simulink model "scale_model_model_control"  (R2024b)
settings: Solver=VariableStepAuto  StartTime=0.0  StopTime=100  MaxStep=0.02  RelTol=1e-3
values from neighbouring files (symbols this model uses):
  A_adrcl = [zeros(N, 1)  eye(N, N) ... (first row only)    [init_scale_blade_suspended_control.m]
  A_ESO_d = [1-l1_ESO_d, delta_t-l1_ESO_d*delta_t, 1/2 * delta_t^2 - 1/2 * l1_ESO_d*delta_t^2 ... (first row only)    [init_scale_blade_suspended_control.m]
  A_MESO_d = A_o_d - l_MESO_d*C_o_d*A_o_d    [init_scale_blade_suspended_control.m]
  b0 = 1.025    [init_scale_blade_suspended_control.m]
  b_adrcl = [zeros(N-1, 1) ... (first row only)    [init_scale_blade_suspended_control.m]
  b_ESO_d = [1/2*b0*delta_t^2 - l1_ESO_d*b0*delta_t^2 ... (first row only)    [init_scale_blade_suspended_control.m]
  B_MESO_d = B_o_d - l_MESO_d*C_o_d*B_o_d    [init_scale_blade_suspended_control.m]
  c_t = [1, zeros(1, N)]    [init_scale_blade_suspended_control.m]
  delta_t = 0.01    [init_scale_blade_suspended_control.m]
  DLADRC_max_effort = 30    [init_scale_blade_suspended_control.m]
  DLQRMADRC_max_effort = 30    [init_scale_blade_suspended_control.m]
  eta_s_init_n = [p_s_init_n;Theta_s_init_n]    [init_scale_blade_suspended_control.m]
  g = 9.81    [init_scale_blade_suspended_control.m]
  inv_M_s = inv(M_s)    [init_scale_blade_suspended_control.m]
  k = ones(N,1)    [init_scale_blade_suspended_control.m]
  k1_c_d = (1 - z_cl)^2/delta_t^2    [init_scale_blade_suspended_control.m]
  k_c_T_dlqr = dlqr(A_m_dlqr,b_m_dlqr,Q,R)    [init_scale_blade_suspended_control.m]
  k_d_T_lqr = (e_m*c_T_d_m_lqr) \ b_m_lqr    [init_scale_blade_suspended_control.m]
  k_s_lqr = -inv(c_T_m_lqr*inv(A_m_lqr-b_m_lqr*k_c_T_lqr)*b_m_lqr)    [init_scale_blade_suspended_control.m]
  k_T_d = [k1_c_d, k2_c_d]    [init_scale_blade_suspended_control.m]
  k_w1_s = gamma * EA/lw1_s_init    (= 19634.9540849)    [init_scale_blade_suspended_control.m]
  k_w2_s = k_w1_s    (= 19634.9540849)    [init_scale_blade_suspended_control.m]
  L = 0.8    [init_scale_blade_suspended_control.m]
  l = ones(N+1, 1)    [init_scale_blade_suspended_control.m]
  l_ESO_d = [l1_ESO_d, l2_ESO_d, l3_ESO_d]'    [init_scale_blade_suspended_control.m]
  l_MESO_d = acker(A_o_d',C_o_d',[z_MESO,z_MESO,z_MESO])'    [init_scale_blade_suspended_control.m]
  lw1_s_init = tot_liftWire-0.14    (= 0.56)    [init_scale_blade_suspended_control.m]
  lw2_s = norm(p_h_s_init- posSling_s_n(:,1))-elong_lw2_s    [init_scale_blade_suspended_control.m]
  m_h_s = 0.01    [init_scale_blade_suspended_control.m]
  meanWSP = 1    [init_scale_blade_suspended_control.m]
  N = 2    [init_scale_blade_suspended_control.m]
  nu_s_init_b = zeros(6,1)    [init_scale_blade_suspended_control.m]
  p_h_dot_s_init = [0;0;0]    [init_scale_blade_suspended_control.m]
  p_h_s_init = posCraneTip_s + [0;0;lw1_s_init + elong_mainlw_s]    [init_scale_blade_suspended_control.m]
  posCOG_s = [0;0;0]    [init_scale_blade_suspended_control.m]
  posCraneTip_s = [0;0;-1.2]    [init_scale_blade_suspended_control.m]
  posSling_s_b = [posCOG_s + [slings_p1_new(1); -0.05; slings_p1_new(2)],                posCOG_s + [slings_p1_new(1); 0.05; slings_p1_new(2)],               posCOG_s + [slings_p2_new(1); -0.05; slings_p2_new(2)],               posCOG_s + [slings_p2_new(1); 0.05; slings_p2_new(2)]]    [init_scale_blade_suspended_control.m]
  posThruster_s_b = [posCOG_s + [0.03; 0.21; -0.05],                posCOG_s + [0.03; -0.21; -0.05],               posCOG_s + [0; 0.1825; -0.05],               posCOG_s + [0; -0.1825; -0.05]]    [init_scale_blade_suspended_control.m]
  totalMass_s = 0.391    [init_scale_blade_suspended_control.m]
  W = 0.05    [init_scale_blade_suspended_control.m]
undefined symbols (not defined in the file or in its folder): A_o_dlqr, b_o_dlqr, c_o_T_dlqr, k_o_lqr, linsys_v2, sigbuilder_block
libraries: MarIn_blade x104, simulink_extras x28, slpidlib x5, simulink x4
(part 3 of 3)

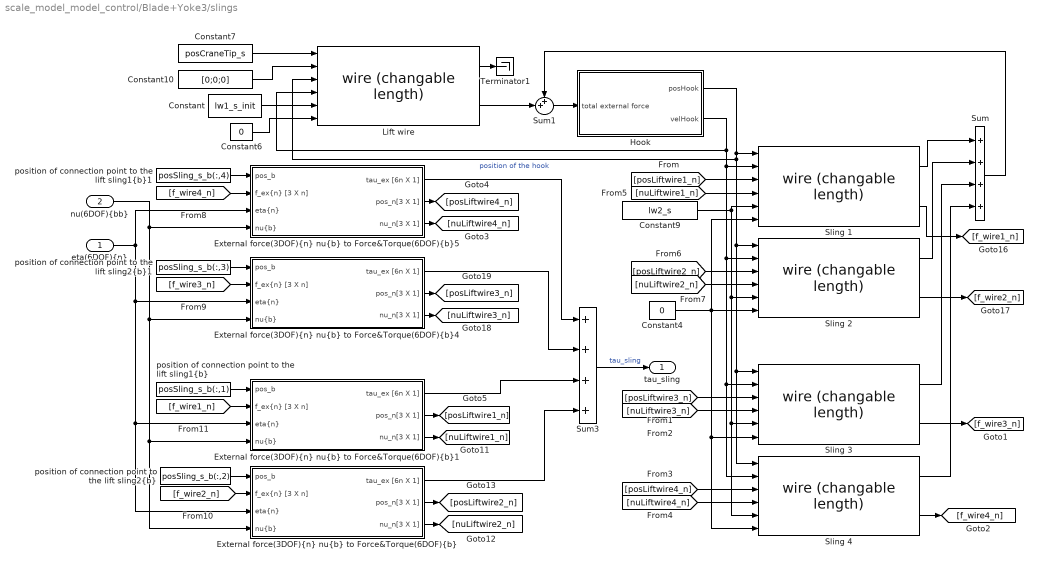
== system scale_model_model_control/Blade+Yoke3/slings ==
  "eta(6DOF){n}" : Inport
  "nu(6DOF){bb}" : Inport  Port=2
  Constant : Constant  Value=lw1_s_init
  Constant10 : Constant  Value=[0;0;0]
  Constant4 : Constant  Value=0
  Constant6 : Constant  Value=0
  Constant7 : Constant  Value=posCraneTip_s
  Constant9 : Constant  Value=lw2_s
  "External force(3DOF){n} nu{b} to Force&Torque(6DOF){b}" : Subsystem  AncestorBlock=MarIn_blade/Basic functions/External force(3DOF){n} nu{b} to Force&Torque(6DOF){b}  mask(External force(3DOF){n} nu{b} to Force&Torque(6DOF){b}){}
      mask help:
      | Translate position and velocity in {b} to {n}.
      |
      |
      | Author: Zhengru Ren
      | Date: April 22, 2017
  "External force(3DOF){n} nu{b} to Force&Torque(6DOF){b}1" : Subsystem  AncestorBlock=MarIn_blade/Basic functions/External force(3DOF){n} nu{b} to Force&Torque(6DOF){b}  mask(External force(3DOF){n} nu{b} to Force&Torque(6DOF){b}){}
      mask help:
      | Translate position and velocity in {b} to {n}.
      |
      |
      | Author: Zhengru Ren
      | Date: April 22, 2017
  "External force(3DOF){n} nu{b} to Force&Torque(6DOF){b}4" : Subsystem  AncestorBlock=MarIn_blade/Basic functions/External force(3DOF){n} nu{b} to Force&Torque(6DOF){b}  mask(External force(3DOF){n} nu{b} to Force&Torque(6DOF){b}){}
      mask help:
      | Translate position and velocity in {b} to {n}.
      |
      |
      | Author: Zhengru Ren
      | Date: April 22, 2017
  "External force(3DOF){n} nu{b} to Force&Torque(6DOF){b}5" : Subsystem  AncestorBlock=MarIn_blade/Basic functions/External force(3DOF){n} nu{b} to Force&Torque(6DOF){b}  mask(External force(3DOF){n} nu{b} to Force&Torque(6DOF){b}){}
      mask help:
      | Translate position and velocity in {b} to {n}.
      |
      |
      | Author: Zhengru Ren
      | Date: April 22, 2017
  Hook : Subsystem  AncestorBlock=|  mask(Hook){m_h=m_h_s, p_h_init=p_h_s_init, p_h_dot_init=p_h_dot_s_init}
      | MarIn_blade/Lifting equipments
      | (winch, wire, hook)/Hook
      mask prompts: m_h "Hook mass (m_h) [kg]"; p_h_init "Initial position of the hook"; p_h_dot_init "Initial velocity of the hook"
      mask help:
      | Used to simulate a hook.
      |
      | Author: Zhengru Ren
      | Date: May 20, 2016
      mask init:
      | invM_h = diag([1/m_h,1/m_h,1/m_h]);
  Lift wire : MarIn_blade/Lifting equipments (winch, wire, hook)/wire (changable length)  k=k_w1_s  c=d_w1_s
      settings: SourceProductName=MarIn (Blade)
  Sling {1..4} (4 alike) : MarIn_blade/Lifting equipments (winch, wire, hook)/wire (changable length)  k=k_w2_s  c=d_w2_s
      settings: SourceProductName=MarIn (Blade)
  Sum : Sum  Inputs=++++
  Sum1 : Sum  Inputs=++|
  Sum3 : Sum  Inputs=4
  Terminator1 : Terminator
  "position of connection point to the lift sling1{b}" : Constant  Value=posSling_s_b(:,1)
  "position of connection point to the lift sling1{b}1" : Constant  Value=posSling_s_b(:,4)
  "position of connection point to the lift sling2{b}" : Constant  Value=posSling_s_b(:,2)
  "position of connection point to the lift sling2{b}1" : Constant  Value=posSling_s_b(:,3)
  tau_sling : Outport
  wires:
  "nu(6DOF){bb}"/1 -> "External force(3DOF){n} nu{b} to Force&Torque(6DOF){b}"/4("nu{b}"), "External force(3DOF){n} nu{b} to Force&Torque(6DOF){b}1"/4("nu{b}"), "External force(3DOF){n} nu{b} to Force&Torque(6DOF){b}4"/4("nu{b}"), "External force(3DOF){n} nu{b} to Force&Torque(6DOF){b}5"/4("nu{b}")
  "position of connection point to the lift sling1{b}1"/1 -> "External force(3DOF){n} nu{b} to Force&Torque(6DOF){b}5"/1(pos_b)
  "External force(3DOF){n} nu{b} to Force&Torque(6DOF){b}"/1(tau_ex [6n X 1]) -> Sum3/4
  "eta(6DOF){n}"/1 -> "External force(3DOF){n} nu{b} to Force&Torque(6DOF){b}5"/3("eta{n}"), "External force(3DOF){n} nu{b} to Force&Torque(6DOF){b}"/3("eta{n}"), "External force(3DOF){n} nu{b} to Force&Torque(6DOF){b}1"/3("eta{n}"), "External force(3DOF){n} nu{b} to Force&Torque(6DOF){b}4"/3("eta{n}")
  "External force(3DOF){n} nu{b} to Force&Torque(6DOF){b}5"/1(tau_ex [6n X 1]) -> Sum3/1
  "position of connection point to the lift sling2{b}"/1 -> "External force(3DOF){n} nu{b} to Force&Torque(6DOF){b}"/1(pos_b)
  Sum3/1 -> tau_sling/1  "tau_sling"
  "External force(3DOF){n} nu{b} to Force&Torque(6DOF){b}4"/1(tau_ex [6n X 1]) -> Sum3/2
  [f_wire4_n] -> "External force(3DOF){n} nu{b} to Force&Torque(6DOF){b}5"/2("f_ex{n} [3 X n]")
  [f_wire3_n] -> "External force(3DOF){n} nu{b} to Force&Torque(6DOF){b}4"/2("f_ex{n} [3 X n]")
  "position of connection point to the lift sling2{b}1"/1 -> "External force(3DOF){n} nu{b} to Force&Torque(6DOF){b}4"/1(pos_b)
  "External force(3DOF){n} nu{b} to Force&Torque(6DOF){b}1"/3(nu_n[3 X 1]) -> [nuLiftwire1_n]
  "External force(3DOF){n} nu{b} to Force&Torque(6DOF){b}4"/2(pos_n[3 X 1]) -> [posLiftwire3_n]
  "position of connection point to the lift sling1{b}"/1 -> "External force(3DOF){n} nu{b} to Force&Torque(6DOF){b}1"/1(pos_b)
  "External force(3DOF){n} nu{b} to Force&Torque(6DOF){b}4"/3(nu_n[3 X 1]) -> [nuLiftwire3_n]
  [f_wire2_n] -> "External force(3DOF){n} nu{b} to Force&Torque(6DOF){b}"/2("f_ex{n} [3 X n]")
  "External force(3DOF){n} nu{b} to Force&Torque(6DOF){b}"/3(nu_n[3 X 1]) -> [nuLiftwire2_n]
  "External force(3DOF){n} nu{b} to Force&Torque(6DOF){b}"/2(pos_n[3 X 1]) -> [posLiftwire2_n]
  "External force(3DOF){n} nu{b} to Force&Torque(6DOF){b}1"/1(tau_ex [6n X 1]) -> Sum3/3
  "External force(3DOF){n} nu{b} to Force&Torque(6DOF){b}1"/2(pos_n[3 X 1]) -> [posLiftwire1_n]
  [f_wire1_n] -> "External force(3DOF){n} nu{b} to Force&Torque(6DOF){b}1"/2("f_ex{n} [3 X n]")
  Sling 4/2 -> [f_wire4_n]
  Sling 3/2 -> [f_wire3_n]
  Sling 4/1 -> Sum/4
  Sling 3/1 -> Sum/3
  [posLiftwire3_n] -> Sling 3/3
  [nuLiftwire3_n] -> Sling 3/4
  Hook/2(velHook) -> Sling 3/2, Sling 4/2, Sling 2/2, Sling 1/2, Lift wire/4
  Constant/1 -> Lift wire/5
  [posLiftwire1_n] -> Sling 1/3
  Sling 1/2 -> [f_wire1_n]
  [nuLiftwire1_n] -> Sling 1/4
  Sling 2/1 -> Sum/2
  Sling 2/2 -> [f_wire2_n]
  [posLiftwire2_n] -> Sling 2/3
  [nuLiftwire2_n] -> Sling 2/4
  Constant9/1 -> Sling 1/5, Sling 2/5, Sling 3/5, Sling 4/5
  Constant7/1 -> Lift wire/1
  Constant10/1 -> Lift wire/2
  Sum/1 -> Sum1/1
  Lift wire/2 -> Sum1/2
  Lift wire/1 -> Terminator1/1
  Sum1/1 -> Hook/1(total external force)
  Hook/1(posHook) -> Sling 3/1, Sling 4/1, Sling 2/1, Lift wire/3, Sling 1/1  "position of the hook"
  Constant4/1 -> Sling 2/6, Sling 1/6, Sling 3/6, Sling 4/6
  Constant6/1 -> Lift wire/6
  Sling 1/1 -> Sum/1
  [nuLiftwire4_n] -> Sling 4/4
  [posLiftwire4_n] -> Sling 4/3
  "External force(3DOF){n} nu{b} to Force&Torque(6DOF){b}5"/3(nu_n[3 X 1]) -> [nuLiftwire4_n]
  "External force(3DOF){n} nu{b} to Force&Torque(6DOF){b}5"/2(pos_n[3 X 1]) -> [posLiftwire4_n]

== system scale_model_model_control/Blade+Yoke3/thrusters ==
  "F_thrusters {b}" : Inport
  Demux : Demux
  Force(3DOF){b}2Force&Torque(6DOF){b}{,1..3} (4 alike) : MarIn_blade/Basic functions/Force(3DOF){b}2Force&Torque(6DOF){b}  posCOG_bb=posCOG_s
      settings: SourceProductName=MarIn (Blade)
  Sum3 : Sum  Inputs=4
  "position of connection point to thruster1{b}" : Constant  Value=posThruster_s_b(:,1)
  "position of connection point to thruster2{b}" : Constant  Value=posThruster_s_b(:,2)
  "position of connection point to thruster3{b}" : Constant  Value=posThruster_s_b(:,3)
  "position of connection point to thruster4{b}" : Constant  Value=posThruster_s_b(:,4)
  tau_thrusters : Outport
  wires:
  "position of connection point to thruster1{b}"/1 -> "Force(3DOF){b}2Force&Torque(6DOF){b}1"/1
  "position of connection point to thruster3{b}"/1 -> "Force(3DOF){b}2Force&Torque(6DOF){b}2"/1
  Sum3/1 -> tau_thrusters/1  "tau_thrusters"
  "position of connection point to thruster2{b}"/1 -> "Force(3DOF){b}2Force&Torque(6DOF){b}"/1
  "Force(3DOF){b}2Force&Torque(6DOF){b}"/1 -> Sum3/4
  "position of connection point to thruster4{b}"/1 -> "Force(3DOF){b}2Force&Torque(6DOF){b}3"/1
  "Force(3DOF){b}2Force&Torque(6DOF){b}3"/1 -> Sum3/1
  "Force(3DOF){b}2Force&Torque(6DOF){b}2"/1 -> Sum3/2
  "Force(3DOF){b}2Force&Torque(6DOF){b}1"/1 -> Sum3/3
  "F_thrusters {b}"/1 -> Demux/1
  Demux/4 -> "Force(3DOF){b}2Force&Torque(6DOF){b}3"/2
  Demux/3 -> "Force(3DOF){b}2Force&Torque(6DOF){b}2"/2
  Demux/1 -> "Force(3DOF){b}2Force&Torque(6DOF){b}1"/2
  Demux/2 -> "Force(3DOF){b}2Force&Torque(6DOF){b}"/2

== system scale_model_model_control/Blade+Yoke/slings/External force(3DOF){n} nu{b} to Force&Torque(6DOF){b} ==
  pos_b : Inport
  "f_ex{n} [3 X n]" : Inport  Port=2
  "eta{n}" : Inport  Port=3
  "nu{b}" : Inport  Port=4
  "Force(3DOF){b}2Force&Torque(6DOF){b}" : MarIn_blade/Basic functions/Force(3DOF){b}2Force&Torque(6DOF){b}  posCOG_bb=posCOG_s
      settings: SourceProductName=MarIn (Blade)
  "Translate velocity&force {n}2{b}" : MarIn_blade/Basic functions/Translate velocity&force {n}2{b}
      settings: SourceProductName=MarIn (Blade)
  "pos{b} nu{b} to pos{n}" : MarIn_blade/Basic functions/pos{b} nu{b} to pos{n}  posCOG_bb=posCOG_s
      settings: SourceProductName=MarIn (Blade)
  tau_ex [6n X 1] : Outport
  pos_n[3 X 1] : Outport  Port=2
  nu_n[3 X 1] : Outport  Port=3
  wires:
  "eta{n}"/1 -> "Translate velocity&force {n}2{b}"/1, "pos{b} nu{b} to pos{n}"/2
  "f_ex{n} [3 X n]"/1 -> "Translate velocity&force {n}2{b}"/2
  "Force(3DOF){b}2Force&Torque(6DOF){b}"/1 -> tau_ex [6n X 1]/1
  "Translate velocity&force {n}2{b}"/1 -> "Force(3DOF){b}2Force&Torque(6DOF){b}"/2  "External force{bb}"
  pos_b/1 -> "Force(3DOF){b}2Force&Torque(6DOF){b}"/1, "pos{b} nu{b} to pos{n}"/1
  "pos{b} nu{b} to pos{n}"/1 -> pos_n[3 X 1]/1
  "nu{b}"/1 -> "pos{b} nu{b} to pos{n}"/3
  "pos{b} nu{b} to pos{n}"/2 -> nu_n[3 X 1]/1

== system scale_model_model_control/Blade+Yoke/slings/External force(3DOF){n} nu{b} to Force&Torque(6DOF){b}1 ==
  pos_b : Inport
  "f_ex{n} [3 X n]" : Inport  Port=2
  "eta{n}" : Inport  Port=3
  "nu{b}" : Inport  Port=4
  "Force(3DOF){b}2Force&Torque(6DOF){b}" : MarIn_blade/Basic functions/Force(3DOF){b}2Force&Torque(6DOF){b}  posCOG_bb=posCOG_s
      settings: SourceProductName=MarIn (Blade)
  "Translate velocity&force {n}2{b}" : MarIn_blade/Basic functions/Translate velocity&force {n}2{b}
      settings: SourceProductName=MarIn (Blade)
  "pos{b} nu{b} to pos{n}" : MarIn_blade/Basic functions/pos{b} nu{b} to pos{n}  posCOG_bb=posCOG_s
      settings: SourceProductName=MarIn (Blade)
  tau_ex [6n X 1] : Outport
  pos_n[3 X 1] : Outport  Port=2
  nu_n[3 X 1] : Outport  Port=3
  wires:
  "eta{n}"/1 -> "Translate velocity&force {n}2{b}"/1, "pos{b} nu{b} to pos{n}"/2
  "f_ex{n} [3 X n]"/1 -> "Translate velocity&force {n}2{b}"/2
  "Force(3DOF){b}2Force&Torque(6DOF){b}"/1 -> tau_ex [6n X 1]/1
  "Translate velocity&force {n}2{b}"/1 -> "Force(3DOF){b}2Force&Torque(6DOF){b}"/2  "External force{bb}"
  pos_b/1 -> "Force(3DOF){b}2Force&Torque(6DOF){b}"/1, "pos{b} nu{b} to pos{n}"/1
  "pos{b} nu{b} to pos{n}"/1 -> pos_n[3 X 1]/1
  "nu{b}"/1 -> "pos{b} nu{b} to pos{n}"/3
  "pos{b} nu{b} to pos{n}"/2 -> nu_n[3 X 1]/1

== system scale_model_model_control/Blade+Yoke/slings/External force(3DOF){n} nu{b} to Force&Torque(6DOF){b}4 ==
  pos_b : Inport
  "f_ex{n} [3 X n]" : Inport  Port=2
  "eta{n}" : Inport  Port=3
  "nu{b}" : Inport  Port=4
  "Force(3DOF){b}2Force&Torque(6DOF){b}" : MarIn_blade/Basic functions/Force(3DOF){b}2Force&Torque(6DOF){b}  posCOG_bb=posCOG_s
      settings: SourceProductName=MarIn (Blade)
  "Translate velocity&force {n}2{b}" : MarIn_blade/Basic functions/Translate velocity&force {n}2{b}
      settings: SourceProductName=MarIn (Blade)
  "pos{b} nu{b} to pos{n}" : MarIn_blade/Basic functions/pos{b} nu{b} to pos{n}  posCOG_bb=posCOG_s
      settings: SourceProductName=MarIn (Blade)
  tau_ex [6n X 1] : Outport
  pos_n[3 X 1] : Outport  Port=2
  nu_n[3 X 1] : Outport  Port=3
  wires:
  "eta{n}"/1 -> "Translate velocity&force {n}2{b}"/1, "pos{b} nu{b} to pos{n}"/2
  "f_ex{n} [3 X n]"/1 -> "Translate velocity&force {n}2{b}"/2
  "Force(3DOF){b}2Force&Torque(6DOF){b}"/1 -> tau_ex [6n X 1]/1
  "Translate velocity&force {n}2{b}"/1 -> "Force(3DOF){b}2Force&Torque(6DOF){b}"/2  "External force{bb}"
  pos_b/1 -> "Force(3DOF){b}2Force&Torque(6DOF){b}"/1, "pos{b} nu{b} to pos{n}"/1
  "pos{b} nu{b} to pos{n}"/1 -> pos_n[3 X 1]/1
  "nu{b}"/1 -> "pos{b} nu{b} to pos{n}"/3
  "pos{b} nu{b} to pos{n}"/2 -> nu_n[3 X 1]/1

== system scale_model_model_control/Blade+Yoke/slings/External force(3DOF){n} nu{b} to Force&Torque(6DOF){b}5 ==
  pos_b : Inport
  "f_ex{n} [3 X n]" : Inport  Port=2
  "eta{n}" : Inport  Port=3
  "nu{b}" : Inport  Port=4
  "Force(3DOF){b}2Force&Torque(6DOF){b}" : MarIn_blade/Basic functions/Force(3DOF){b}2Force&Torque(6DOF){b}  posCOG_bb=posCOG_s
      settings: SourceProductName=MarIn (Blade)
  "Translate velocity&force {n}2{b}" : MarIn_blade/Basic functions/Translate velocity&force {n}2{b}
      settings: SourceProductName=MarIn (Blade)
  "pos{b} nu{b} to pos{n}" : MarIn_blade/Basic functions/pos{b} nu{b} to pos{n}  posCOG_bb=posCOG_s
      settings: SourceProductName=MarIn (Blade)
  tau_ex [6n X 1] : Outport
  pos_n[3 X 1] : Outport  Port=2
  nu_n[3 X 1] : Outport  Port=3
  wires:
  "eta{n}"/1 -> "Translate velocity&force {n}2{b}"/1, "pos{b} nu{b} to pos{n}"/2
  "f_ex{n} [3 X n]"/1 -> "Translate velocity&force {n}2{b}"/2
  "Force(3DOF){b}2Force&Torque(6DOF){b}"/1 -> tau_ex [6n X 1]/1
  "Translate velocity&force {n}2{b}"/1 -> "Force(3DOF){b}2Force&Torque(6DOF){b}"/2  "External force{bb}"
  pos_b/1 -> "Force(3DOF){b}2Force&Torque(6DOF){b}"/1, "pos{b} nu{b} to pos{n}"/1
  "pos{b} nu{b} to pos{n}"/1 -> pos_n[3 X 1]/1
  "nu{b}"/1 -> "pos{b} nu{b} to pos{n}"/3
  "pos{b} nu{b} to pos{n}"/2 -> nu_n[3 X 1]/1

== system scale_model_model_control/Blade+Yoke/slings/Hook ==
  total external force : Inport
  Integrator2 : Integrator  InitialCondition=p_h_dot_init  ContinuousStateAttributes='nu_hook'
  Integrator3 : Integrator  InitialCondition=p_h_init  ContinuousStateAttributes='pos_hook'
  Sum6 : Sum
  hook gravity : Constant  Value=[0;0;m_h*g]
  invM_h : Gain  Gain=invM_h  Multiplication=Matrix(K*u)
  posHook : Outport
  velHook : Outport  Port=2
  wires:
  Integrator2/1 -> velHook/1, Integrator3/1  "p_h_dot"
  total external force/1 -> Sum6/1
  hook gravity/1 -> Sum6/2
  invM_h/1 -> Integrator2/1  "p_h_ddot"
  Sum6/1 -> invM_h/1
  Integrator3/1 -> posHook/1  "p_h"

== system scale_model_model_control/Blade+Yoke1/slings/External force(3DOF){n} nu{b} to Force&Torque(6DOF){b} ==
  pos_b : Inport
  "f_ex{n} [3 X n]" : Inport  Port=2
  "eta{n}" : Inport  Port=3
  "nu{b}" : Inport  Port=4
  "Force(3DOF){b}2Force&Torque(6DOF){b}" : MarIn_blade/Basic functions/Force(3DOF){b}2Force&Torque(6DOF){b}  posCOG_bb=posCOG_s
      settings: SourceProductName=MarIn (Blade)
  "Translate velocity&force {n}2{b}" : MarIn_blade/Basic functions/Translate velocity&force {n}2{b}
      settings: SourceProductName=MarIn (Blade)
  "pos{b} nu{b} to pos{n}" : MarIn_blade/Basic functions/pos{b} nu{b} to pos{n}  posCOG_bb=posCOG_s
      settings: SourceProductName=MarIn (Blade)
  tau_ex [6n X 1] : Outport
  pos_n[3 X 1] : Outport  Port=2
  nu_n[3 X 1] : Outport  Port=3
  wires:
  "eta{n}"/1 -> "Translate velocity&force {n}2{b}"/1, "pos{b} nu{b} to pos{n}"/2
  "f_ex{n} [3 X n]"/1 -> "Translate velocity&force {n}2{b}"/2
  "Force(3DOF){b}2Force&Torque(6DOF){b}"/1 -> tau_ex [6n X 1]/1
  "Translate velocity&force {n}2{b}"/1 -> "Force(3DOF){b}2Force&Torque(6DOF){b}"/2  "External force{bb}"
  pos_b/1 -> "Force(3DOF){b}2Force&Torque(6DOF){b}"/1, "pos{b} nu{b} to pos{n}"/1
  "pos{b} nu{b} to pos{n}"/1 -> pos_n[3 X 1]/1
  "nu{b}"/1 -> "pos{b} nu{b} to pos{n}"/3
  "pos{b} nu{b} to pos{n}"/2 -> nu_n[3 X 1]/1

== system scale_model_model_control/Blade+Yoke1/slings/External force(3DOF){n} nu{b} to Force&Torque(6DOF){b}1 ==
  pos_b : Inport
  "f_ex{n} [3 X n]" : Inport  Port=2
  "eta{n}" : Inport  Port=3
  "nu{b}" : Inport  Port=4
  "Force(3DOF){b}2Force&Torque(6DOF){b}" : MarIn_blade/Basic functions/Force(3DOF){b}2Force&Torque(6DOF){b}  posCOG_bb=posCOG_s
      settings: SourceProductName=MarIn (Blade)
  "Translate velocity&force {n}2{b}" : MarIn_blade/Basic functions/Translate velocity&force {n}2{b}
      settings: SourceProductName=MarIn (Blade)
  "pos{b} nu{b} to pos{n}" : MarIn_blade/Basic functions/pos{b} nu{b} to pos{n}  posCOG_bb=posCOG_s
      settings: SourceProductName=MarIn (Blade)
  tau_ex [6n X 1] : Outport
  pos_n[3 X 1] : Outport  Port=2
  nu_n[3 X 1] : Outport  Port=3
  wires:
  "eta{n}"/1 -> "Translate velocity&force {n}2{b}"/1, "pos{b} nu{b} to pos{n}"/2
  "f_ex{n} [3 X n]"/1 -> "Translate velocity&force {n}2{b}"/2
  "Force(3DOF){b}2Force&Torque(6DOF){b}"/1 -> tau_ex [6n X 1]/1
  "Translate velocity&force {n}2{b}"/1 -> "Force(3DOF){b}2Force&Torque(6DOF){b}"/2  "External force{bb}"
  pos_b/1 -> "Force(3DOF){b}2Force&Torque(6DOF){b}"/1, "pos{b} nu{b} to pos{n}"/1
  "pos{b} nu{b} to pos{n}"/1 -> pos_n[3 X 1]/1
  "nu{b}"/1 -> "pos{b} nu{b} to pos{n}"/3
  "pos{b} nu{b} to pos{n}"/2 -> nu_n[3 X 1]/1

== system scale_model_model_control/Blade+Yoke1/slings/External force(3DOF){n} nu{b} to Force&Torque(6DOF){b}4 ==
  pos_b : Inport
  "f_ex{n} [3 X n]" : Inport  Port=2
  "eta{n}" : Inport  Port=3
  "nu{b}" : Inport  Port=4
  "Force(3DOF){b}2Force&Torque(6DOF){b}" : MarIn_blade/Basic functions/Force(3DOF){b}2Force&Torque(6DOF){b}  posCOG_bb=posCOG_s
      settings: SourceProductName=MarIn (Blade)
  "Translate velocity&force {n}2{b}" : MarIn_blade/Basic functions/Translate velocity&force {n}2{b}
      settings: SourceProductName=MarIn (Blade)
  "pos{b} nu{b} to pos{n}" : MarIn_blade/Basic functions/pos{b} nu{b} to pos{n}  posCOG_bb=posCOG_s
      settings: SourceProductName=MarIn (Blade)
  tau_ex [6n X 1] : Outport
  pos_n[3 X 1] : Outport  Port=2
  nu_n[3 X 1] : Outport  Port=3
  wires:
  "eta{n}"/1 -> "Translate velocity&force {n}2{b}"/1, "pos{b} nu{b} to pos{n}"/2
  "f_ex{n} [3 X n]"/1 -> "Translate velocity&force {n}2{b}"/2
  "Force(3DOF){b}2Force&Torque(6DOF){b}"/1 -> tau_ex [6n X 1]/1
  "Translate velocity&force {n}2{b}"/1 -> "Force(3DOF){b}2Force&Torque(6DOF){b}"/2  "External force{bb}"
  pos_b/1 -> "Force(3DOF){b}2Force&Torque(6DOF){b}"/1, "pos{b} nu{b} to pos{n}"/1
  "pos{b} nu{b} to pos{n}"/1 -> pos_n[3 X 1]/1
  "nu{b}"/1 -> "pos{b} nu{b} to pos{n}"/3
  "pos{b} nu{b} to pos{n}"/2 -> nu_n[3 X 1]/1

== system scale_model_model_control/Blade+Yoke1/slings/External force(3DOF){n} nu{b} to Force&Torque(6DOF){b}5 ==
  pos_b : Inport
  "f_ex{n} [3 X n]" : Inport  Port=2
  "eta{n}" : Inport  Port=3
  "nu{b}" : Inport  Port=4
  "Force(3DOF){b}2Force&Torque(6DOF){b}" : MarIn_blade/Basic functions/Force(3DOF){b}2Force&Torque(6DOF){b}  posCOG_bb=posCOG_s
      settings: SourceProductName=MarIn (Blade)
  "Translate velocity&force {n}2{b}" : MarIn_blade/Basic functions/Translate velocity&force {n}2{b}
      settings: SourceProductName=MarIn (Blade)
  "pos{b} nu{b} to pos{n}" : MarIn_blade/Basic functions/pos{b} nu{b} to pos{n}  posCOG_bb=posCOG_s
      settings: SourceProductName=MarIn (Blade)
  tau_ex [6n X 1] : Outport
  pos_n[3 X 1] : Outport  Port=2
  nu_n[3 X 1] : Outport  Port=3
  wires:
  "eta{n}"/1 -> "Translate velocity&force {n}2{b}"/1, "pos{b} nu{b} to pos{n}"/2
  "f_ex{n} [3 X n]"/1 -> "Translate velocity&force {n}2{b}"/2
  "Force(3DOF){b}2Force&Torque(6DOF){b}"/1 -> tau_ex [6n X 1]/1
  "Translate velocity&force {n}2{b}"/1 -> "Force(3DOF){b}2Force&Torque(6DOF){b}"/2  "External force{bb}"
  pos_b/1 -> "Force(3DOF){b}2Force&Torque(6DOF){b}"/1, "pos{b} nu{b} to pos{n}"/1
  "pos{b} nu{b} to pos{n}"/1 -> pos_n[3 X 1]/1
  "nu{b}"/1 -> "pos{b} nu{b} to pos{n}"/3
  "pos{b} nu{b} to pos{n}"/2 -> nu_n[3 X 1]/1

== system scale_model_model_control/Blade+Yoke1/slings/Hook ==
  total external force : Inport
  Integrator2 : Integrator  InitialCondition=p_h_dot_init  ContinuousStateAttributes='nu_hook'
  Integrator3 : Integrator  InitialCondition=p_h_init  ContinuousStateAttributes='pos_hook'
  Sum6 : Sum
  hook gravity : Constant  Value=[0;0;m_h*g]
  invM_h : Gain  Gain=invM_h  Multiplication=Matrix(K*u)
  posHook : Outport
  velHook : Outport  Port=2
  wires:
  Integrator2/1 -> velHook/1, Integrator3/1  "p_h_dot"
  total external force/1 -> Sum6/1
  hook gravity/1 -> Sum6/2
  invM_h/1 -> Integrator2/1  "p_h_ddot"
  Sum6/1 -> invM_h/1
  Integrator3/1 -> posHook/1  "p_h"

== system scale_model_model_control/Blade+Yoke2/slings/External force(3DOF){n} nu{b} to Force&Torque(6DOF){b} ==
  pos_b : Inport
  "f_ex{n} [3 X n]" : Inport  Port=2
  "eta{n}" : Inport  Port=3
  "nu{b}" : Inport  Port=4
  "Force(3DOF){b}2Force&Torque(6DOF){b}" : MarIn_blade/Basic functions/Force(3DOF){b}2Force&Torque(6DOF){b}  posCOG_bb=posCOG_s
      settings: SourceProductName=MarIn (Blade)
  "Translate velocity&force {n}2{b}" : MarIn_blade/Basic functions/Translate velocity&force {n}2{b}
      settings: SourceProductName=MarIn (Blade)
  "pos{b} nu{b} to pos{n}" : MarIn_blade/Basic functions/pos{b} nu{b} to pos{n}  posCOG_bb=posCOG_s
      settings: SourceProductName=MarIn (Blade)
  tau_ex [6n X 1] : Outport
  pos_n[3 X 1] : Outport  Port=2
  nu_n[3 X 1] : Outport  Port=3
  wires:
  "eta{n}"/1 -> "Translate velocity&force {n}2{b}"/1, "pos{b} nu{b} to pos{n}"/2
  "f_ex{n} [3 X n]"/1 -> "Translate velocity&force {n}2{b}"/2
  "Force(3DOF){b}2Force&Torque(6DOF){b}"/1 -> tau_ex [6n X 1]/1
  "Translate velocity&force {n}2{b}"/1 -> "Force(3DOF){b}2Force&Torque(6DOF){b}"/2  "External force{bb}"
  pos_b/1 -> "Force(3DOF){b}2Force&Torque(6DOF){b}"/1, "pos{b} nu{b} to pos{n}"/1
  "pos{b} nu{b} to pos{n}"/1 -> pos_n[3 X 1]/1
  "nu{b}"/1 -> "pos{b} nu{b} to pos{n}"/3
  "pos{b} nu{b} to pos{n}"/2 -> nu_n[3 X 1]/1

== system scale_model_model_control/Blade+Yoke2/slings/External force(3DOF){n} nu{b} to Force&Torque(6DOF){b}1 ==
  pos_b : Inport
  "f_ex{n} [3 X n]" : Inport  Port=2
  "eta{n}" : Inport  Port=3
  "nu{b}" : Inport  Port=4
  "Force(3DOF){b}2Force&Torque(6DOF){b}" : MarIn_blade/Basic functions/Force(3DOF){b}2Force&Torque(6DOF){b}  posCOG_bb=posCOG_s
      settings: SourceProductName=MarIn (Blade)
  "Translate velocity&force {n}2{b}" : MarIn_blade/Basic functions/Translate velocity&force {n}2{b}
      settings: SourceProductName=MarIn (Blade)
  "pos{b} nu{b} to pos{n}" : MarIn_blade/Basic functions/pos{b} nu{b} to pos{n}  posCOG_bb=posCOG_s
      settings: SourceProductName=MarIn (Blade)
  tau_ex [6n X 1] : Outport
  pos_n[3 X 1] : Outport  Port=2
  nu_n[3 X 1] : Outport  Port=3
  wires:
  "eta{n}"/1 -> "Translate velocity&force {n}2{b}"/1, "pos{b} nu{b} to pos{n}"/2
  "f_ex{n} [3 X n]"/1 -> "Translate velocity&force {n}2{b}"/2
  "Force(3DOF){b}2Force&Torque(6DOF){b}"/1 -> tau_ex [6n X 1]/1
  "Translate velocity&force {n}2{b}"/1 -> "Force(3DOF){b}2Force&Torque(6DOF){b}"/2  "External force{bb}"
  pos_b/1 -> "Force(3DOF){b}2Force&Torque(6DOF){b}"/1, "pos{b} nu{b} to pos{n}"/1
  "pos{b} nu{b} to pos{n}"/1 -> pos_n[3 X 1]/1
  "nu{b}"/1 -> "pos{b} nu{b} to pos{n}"/3
  "pos{b} nu{b} to pos{n}"/2 -> nu_n[3 X 1]/1

== system scale_model_model_control/Blade+Yoke2/slings/External force(3DOF){n} nu{b} to Force&Torque(6DOF){b}4 ==
  pos_b : Inport
  "f_ex{n} [3 X n]" : Inport  Port=2
  "eta{n}" : Inport  Port=3
  "nu{b}" : Inport  Port=4
  "Force(3DOF){b}2Force&Torque(6DOF){b}" : MarIn_blade/Basic functions/Force(3DOF){b}2Force&Torque(6DOF){b}  posCOG_bb=posCOG_s
      settings: SourceProductName=MarIn (Blade)
  "Translate velocity&force {n}2{b}" : MarIn_blade/Basic functions/Translate velocity&force {n}2{b}
      settings: SourceProductName=MarIn (Blade)
  "pos{b} nu{b} to pos{n}" : MarIn_blade/Basic functions/pos{b} nu{b} to pos{n}  posCOG_bb=posCOG_s
      settings: SourceProductName=MarIn (Blade)
  tau_ex [6n X 1] : Outport
  pos_n[3 X 1] : Outport  Port=2
  nu_n[3 X 1] : Outport  Port=3
  wires:
  "eta{n}"/1 -> "Translate velocity&force {n}2{b}"/1, "pos{b} nu{b} to pos{n}"/2
  "f_ex{n} [3 X n]"/1 -> "Translate velocity&force {n}2{b}"/2
  "Force(3DOF){b}2Force&Torque(6DOF){b}"/1 -> tau_ex [6n X 1]/1
  "Translate velocity&force {n}2{b}"/1 -> "Force(3DOF){b}2Force&Torque(6DOF){b}"/2  "External force{bb}"
  pos_b/1 -> "Force(3DOF){b}2Force&Torque(6DOF){b}"/1, "pos{b} nu{b} to pos{n}"/1
  "pos{b} nu{b} to pos{n}"/1 -> pos_n[3 X 1]/1
  "nu{b}"/1 -> "pos{b} nu{b} to pos{n}"/3
  "pos{b} nu{b} to pos{n}"/2 -> nu_n[3 X 1]/1

== system scale_model_model_control/Blade+Yoke2/slings/External force(3DOF){n} nu{b} to Force&Torque(6DOF){b}5 ==
  pos_b : Inport
  "f_ex{n} [3 X n]" : Inport  Port=2
  "eta{n}" : Inport  Port=3
  "nu{b}" : Inport  Port=4
  "Force(3DOF){b}2Force&Torque(6DOF){b}" : MarIn_blade/Basic functions/Force(3DOF){b}2Force&Torque(6DOF){b}  posCOG_bb=posCOG_s
      settings: SourceProductName=MarIn (Blade)
  "Translate velocity&force {n}2{b}" : MarIn_blade/Basic functions/Translate velocity&force {n}2{b}
      settings: SourceProductName=MarIn (Blade)
  "pos{b} nu{b} to pos{n}" : MarIn_blade/Basic functions/pos{b} nu{b} to pos{n}  posCOG_bb=posCOG_s
      settings: SourceProductName=MarIn (Blade)
  tau_ex [6n X 1] : Outport
  pos_n[3 X 1] : Outport  Port=2
  nu_n[3 X 1] : Outport  Port=3
  wires:
  "eta{n}"/1 -> "Translate velocity&force {n}2{b}"/1, "pos{b} nu{b} to pos{n}"/2
  "f_ex{n} [3 X n]"/1 -> "Translate velocity&force {n}2{b}"/2
  "Force(3DOF){b}2Force&Torque(6DOF){b}"/1 -> tau_ex [6n X 1]/1
  "Translate velocity&force {n}2{b}"/1 -> "Force(3DOF){b}2Force&Torque(6DOF){b}"/2  "External force{bb}"
  pos_b/1 -> "Force(3DOF){b}2Force&Torque(6DOF){b}"/1, "pos{b} nu{b} to pos{n}"/1
  "pos{b} nu{b} to pos{n}"/1 -> pos_n[3 X 1]/1
  "nu{b}"/1 -> "pos{b} nu{b} to pos{n}"/3
  "pos{b} nu{b} to pos{n}"/2 -> nu_n[3 X 1]/1

== system scale_model_model_control/Blade+Yoke2/slings/Hook ==
  total external force : Inport
  Integrator2 : Integrator  InitialCondition=p_h_dot_init  ContinuousStateAttributes='nu_hook'
  Integrator3 : Integrator  InitialCondition=p_h_init  ContinuousStateAttributes='pos_hook'
  Sum6 : Sum
  hook gravity : Constant  Value=[0;0;m_h*g]
  invM_h : Gain  Gain=invM_h  Multiplication=Matrix(K*u)
  posHook : Outport
  velHook : Outport  Port=2
  wires:
  Integrator2/1 -> velHook/1, Integrator3/1  "p_h_dot"
  total external force/1 -> Sum6/1
  hook gravity/1 -> Sum6/2
  invM_h/1 -> Integrator2/1  "p_h_ddot"
  Sum6/1 -> invM_h/1
  Integrator3/1 -> posHook/1  "p_h"

== system scale_model_model_control/Blade+Yoke3/slings/External force(3DOF){n} nu{b} to Force&Torque(6DOF){b} ==
  pos_b : Inport
  "f_ex{n} [3 X n]" : Inport  Port=2
  "eta{n}" : Inport  Port=3
  "nu{b}" : Inport  Port=4
  "Force(3DOF){b}2Force&Torque(6DOF){b}" : MarIn_blade/Basic functions/Force(3DOF){b}2Force&Torque(6DOF){b}  posCOG_bb=posCOG_s
      settings: SourceProductName=MarIn (Blade)
  "Translate velocity&force {n}2{b}" : MarIn_blade/Basic functions/Translate velocity&force {n}2{b}
      settings: SourceProductName=MarIn (Blade)
  "pos{b} nu{b} to pos{n}" : MarIn_blade/Basic functions/pos{b} nu{b} to pos{n}  posCOG_bb=posCOG_s
      settings: SourceProductName=MarIn (Blade)
  tau_ex [6n X 1] : Outport
  pos_n[3 X 1] : Outport  Port=2
  nu_n[3 X 1] : Outport  Port=3
  wires:
  "eta{n}"/1 -> "Translate velocity&force {n}2{b}"/1, "pos{b} nu{b} to pos{n}"/2
  "f_ex{n} [3 X n]"/1 -> "Translate velocity&force {n}2{b}"/2
  "Force(3DOF){b}2Force&Torque(6DOF){b}"/1 -> tau_ex [6n X 1]/1
  "Translate velocity&force {n}2{b}"/1 -> "Force(3DOF){b}2Force&Torque(6DOF){b}"/2  "External force{bb}"
  pos_b/1 -> "Force(3DOF){b}2Force&Torque(6DOF){b}"/1, "pos{b} nu{b} to pos{n}"/1
  "pos{b} nu{b} to pos{n}"/1 -> pos_n[3 X 1]/1
  "nu{b}"/1 -> "pos{b} nu{b} to pos{n}"/3
  "pos{b} nu{b} to pos{n}"/2 -> nu_n[3 X 1]/1

== system scale_model_model_control/Blade+Yoke3/slings/External force(3DOF){n} nu{b} to Force&Torque(6DOF){b}1 ==
  pos_b : Inport
  "f_ex{n} [3 X n]" : Inport  Port=2
  "eta{n}" : Inport  Port=3
  "nu{b}" : Inport  Port=4
  "Force(3DOF){b}2Force&Torque(6DOF){b}" : MarIn_blade/Basic functions/Force(3DOF){b}2Force&Torque(6DOF){b}  posCOG_bb=posCOG_s
      settings: SourceProductName=MarIn (Blade)
  "Translate velocity&force {n}2{b}" : MarIn_blade/Basic functions/Translate velocity&force {n}2{b}
      settings: SourceProductName=MarIn (Blade)
  "pos{b} nu{b} to pos{n}" : MarIn_blade/Basic functions/pos{b} nu{b} to pos{n}  posCOG_bb=posCOG_s
      settings: SourceProductName=MarIn (Blade)
  tau_ex [6n X 1] : Outport
  pos_n[3 X 1] : Outport  Port=2
  nu_n[3 X 1] : Outport  Port=3
  wires:
  "eta{n}"/1 -> "Translate velocity&force {n}2{b}"/1, "pos{b} nu{b} to pos{n}"/2
  "f_ex{n} [3 X n]"/1 -> "Translate velocity&force {n}2{b}"/2
  "Force(3DOF){b}2Force&Torque(6DOF){b}"/1 -> tau_ex [6n X 1]/1
  "Translate velocity&force {n}2{b}"/1 -> "Force(3DOF){b}2Force&Torque(6DOF){b}"/2  "External force{bb}"
  pos_b/1 -> "Force(3DOF){b}2Force&Torque(6DOF){b}"/1, "pos{b} nu{b} to pos{n}"/1
  "pos{b} nu{b} to pos{n}"/1 -> pos_n[3 X 1]/1
  "nu{b}"/1 -> "pos{b} nu{b} to pos{n}"/3
  "pos{b} nu{b} to pos{n}"/2 -> nu_n[3 X 1]/1

== system scale_model_model_control/Blade+Yoke3/slings/External force(3DOF){n} nu{b} to Force&Torque(6DOF){b}4 ==
  pos_b : Inport
  "f_ex{n} [3 X n]" : Inport  Port=2
  "eta{n}" : Inport  Port=3
  "nu{b}" : Inport  Port=4
  "Force(3DOF){b}2Force&Torque(6DOF){b}" : MarIn_blade/Basic functions/Force(3DOF){b}2Force&Torque(6DOF){b}  posCOG_bb=posCOG_s
      settings: SourceProductName=MarIn (Blade)
  "Translate velocity&force {n}2{b}" : MarIn_blade/Basic functions/Translate velocity&force {n}2{b}
      settings: SourceProductName=MarIn (Blade)
  "pos{b} nu{b} to pos{n}" : MarIn_blade/Basic functions/pos{b} nu{b} to pos{n}  posCOG_bb=posCOG_s
      settings: SourceProductName=MarIn (Blade)
  tau_ex [6n X 1] : Outport
  pos_n[3 X 1] : Outport  Port=2
  nu_n[3 X 1] : Outport  Port=3
  wires:
  "eta{n}"/1 -> "Translate velocity&force {n}2{b}"/1, "pos{b} nu{b} to pos{n}"/2
  "f_ex{n} [3 X n]"/1 -> "Translate velocity&force {n}2{b}"/2
  "Force(3DOF){b}2Force&Torque(6DOF){b}"/1 -> tau_ex [6n X 1]/1
  "Translate velocity&force {n}2{b}"/1 -> "Force(3DOF){b}2Force&Torque(6DOF){b}"/2  "External force{bb}"
  pos_b/1 -> "Force(3DOF){b}2Force&Torque(6DOF){b}"/1, "pos{b} nu{b} to pos{n}"/1
  "pos{b} nu{b} to pos{n}"/1 -> pos_n[3 X 1]/1
  "nu{b}"/1 -> "pos{b} nu{b} to pos{n}"/3
  "pos{b} nu{b} to pos{n}"/2 -> nu_n[3 X 1]/1

== system scale_model_model_control/Blade+Yoke3/slings/External force(3DOF){n} nu{b} to Force&Torque(6DOF){b}5 ==
  pos_b : Inport
  "f_ex{n} [3 X n]" : Inport  Port=2
  "eta{n}" : Inport  Port=3
  "nu{b}" : Inport  Port=4
  "Force(3DOF){b}2Force&Torque(6DOF){b}" : MarIn_blade/Basic functions/Force(3DOF){b}2Force&Torque(6DOF){b}  posCOG_bb=posCOG_s
      settings: SourceProductName=MarIn (Blade)
  "Translate velocity&force {n}2{b}" : MarIn_blade/Basic functions/Translate velocity&force {n}2{b}
      settings: SourceProductName=MarIn (Blade)
  "pos{b} nu{b} to pos{n}" : MarIn_blade/Basic functions/pos{b} nu{b} to pos{n}  posCOG_bb=posCOG_s
      settings: SourceProductName=MarIn (Blade)
  tau_ex [6n X 1] : Outport
  pos_n[3 X 1] : Outport  Port=2
  nu_n[3 X 1] : Outport  Port=3
  wires:
  "eta{n}"/1 -> "Translate velocity&force {n}2{b}"/1, "pos{b} nu{b} to pos{n}"/2
  "f_ex{n} [3 X n]"/1 -> "Translate velocity&force {n}2{b}"/2
  "Force(3DOF){b}2Force&Torque(6DOF){b}"/1 -> tau_ex [6n X 1]/1
  "Translate velocity&force {n}2{b}"/1 -> "Force(3DOF){b}2Force&Torque(6DOF){b}"/2  "External force{bb}"
  pos_b/1 -> "Force(3DOF){b}2Force&Torque(6DOF){b}"/1, "pos{b} nu{b} to pos{n}"/1
  "pos{b} nu{b} to pos{n}"/1 -> pos_n[3 X 1]/1
  "nu{b}"/1 -> "pos{b} nu{b} to pos{n}"/3
  "pos{b} nu{b} to pos{n}"/2 -> nu_n[3 X 1]/1

== system scale_model_model_control/Blade+Yoke3/slings/Hook ==
  total external force : Inport
  Integrator2 : Integrator  InitialCondition=p_h_dot_init  ContinuousStateAttributes='nu_hook'
  Integrator3 : Integrator  InitialCondition=p_h_init  ContinuousStateAttributes='pos_hook'
  Sum6 : Sum
  hook gravity : Constant  Value=[0;0;m_h*g]
  invM_h : Gain  Gain=invM_h  Multiplication=Matrix(K*u)
  posHook : Outport
  velHook : Outport  Port=2
  wires:
  Integrator2/1 -> velHook/1, Integrator3/1  "p_h_dot"
  total external force/1 -> Sum6/1
  hook gravity/1 -> Sum6/2
  invM_h/1 -> Integrator2/1  "p_h_ddot"
  Sum6/1 -> invM_h/1
  Integrator3/1 -> posHook/1  "p_h"
